simulink model "ConverterControl"  (R2024a)
settings: Solver=FixedStepAuto  StartTime=0.0  StopTime=10.0  FixedStep=0.0001  RelTol=1e-3
model workspace (MAT data in the model file):
  Ts = 0.001
libraries: slpidlib x1
settings Model: Creator=Henrique Mesquita  LastModifiedBy=Henrique Mesquita
settings ModelReferenceCC: EnableParallelModelReferenceBuilds=on  ParallelModelReferenceMATLABWorkerInit=Load Top Model

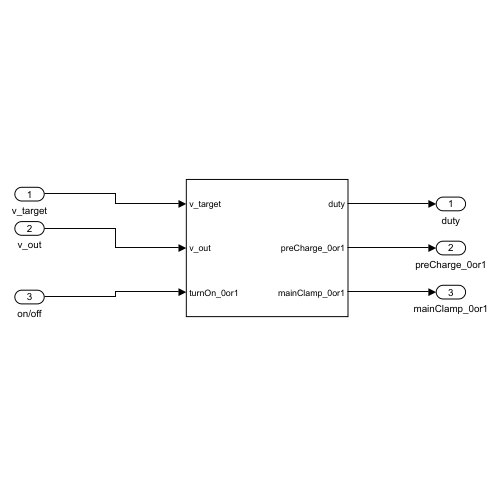
[thumbnail: Simulink's stored preview of the top-level diagram]
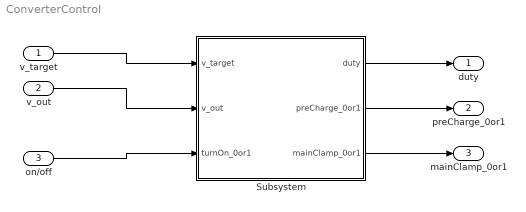
== system ConverterControl ==
  v_target : Inport
  v_out : Inport  Port=2
  on/off : Inport  Port=3
  Subsystem : Subsystem
  duty : Outport
  preCharge_0or1 : Outport  Port=2
  mainClamp_0or1 : Outport  Port=3
  wires:
  v_target/1 -> Subsystem/1(v_target)
  v_out/1 -> Subsystem/2(v_out)
  on/off/1 -> Subsystem/3(turnOn_0or1)
  Subsystem/1(duty) -> duty/1
  Subsystem/2(preCharge_0or1) -> preCharge_0or1/1
  Subsystem/3(mainClamp_0or1) -> mainClamp_0or1/1

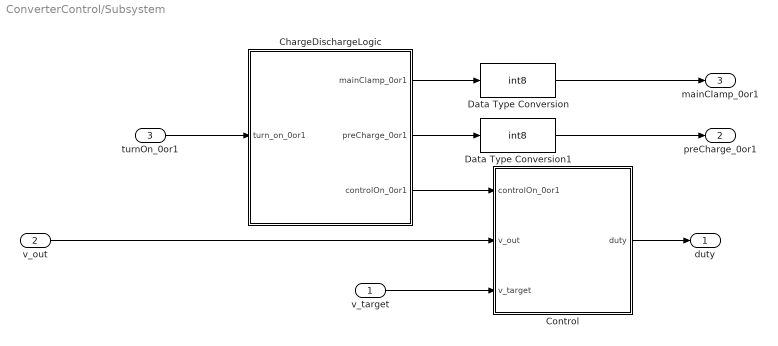
== system ConverterControl/Subsystem ==
  v_target : Inport
  v_out : Inport  Port=2
  turnOn_0or1 : Inport  Port=3
  ChargeDischargeLogic : Stateflow chart  TreatAsAtomicUnit=on
      settings: MinAlgLoopOccurrences=on  PortSchema="{\"entries\":[{\"content\":{\"sides\":[{\"content\":{\"connectorIds\":[\"In1\"]},\"type\":\"ConnectorPlacement.EquallySpacedRectSide\",\"uuid\":\"910d4061-f626-4e59-a733-d82b97cff3cc\"},{\"content\":{\"connectorIds\":[\"Out2\",\"Out3\",\"Out1\"],\"side\":\"RIGHT\"},\"type\":\"ConnectorPlacement.EquallySpacedRectSide\",\"uuid\":\"b59b9408-6f77-4dbd-8f13-72437fb6cf18\"},{\"content\":{\"side\":\"TOP\"},\"type\":\"ConnectorPlacement.EquallySpacedRectSide\",\"uuid\":\"cf8d6f90-ecc3-4087-bd33-4c97bca352fd\"}]},\"type\":\"ConnectorPlacement.EquallySpacedConnector\",\"uuid\":\"df8521dc-5e97-4acd-b29d-9728290d2892\"}],\"packageUris\":[\"http://schema.mathworks.com/mf0/Connector/R2020b\"],\"version\":\"1.0\"}"
  Control : Subsystem
  Data Type Conversion : DataTypeConversion  OutDataTypeStr=int8  SaturateOnIntegerOverflow=off  RndMeth=Floor
  Data Type Conversion1 : DataTypeConversion  OutDataTypeStr=int8  SaturateOnIntegerOverflow=off  RndMeth=Floor
  duty : Outport
  preCharge_0or1 : Outport  Port=2  OutDataTypeStr=int8
  mainClamp_0or1 : Outport  Port=3  OutDataTypeStr=int8
  wires:
  v_target/1 -> Control/3(v_target)
  v_out/1 -> Control/2(v_out)
  ChargeDischargeLogic/1(controlOn_0or1) -> Control/1(controlOn_0or1)
  Control/1(duty) -> duty/1
  turnOn_0or1/1 -> ChargeDischargeLogic/1(turn_on_0or1)
  ChargeDischargeLogic/3(preCharge_0or1) -> Data Type Conversion1/1
  ChargeDischargeLogic/2(mainClamp_0or1) -> Data Type Conversion/1
  Data Type Conversion/1 -> mainClamp_0or1/1
  Data Type Conversion1/1 -> preCharge_0or1/1

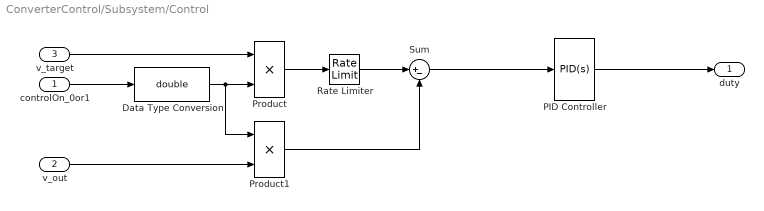
== system ConverterControl/Subsystem/Control ==
  controlOn_0or1 : Inport
  v_out : Inport  Port=2
  v_target : Inport  Port=3
  Data Type Conversion : DataTypeConversion  OutDataTypeStr=double  SaturateOnIntegerOverflow=off  RndMeth=Floor
  PID Controller : slpidlib/PID Controller  Controller=PID  Form=Parallel  TimeDomain=Continuous-time  UseExternalTs=off  SampleTime=-1  IntegratorMethod=Forward Euler  FilterMethod=Forward Euler  ControllerParametersSource=internal  P=0.000137  I=0.512  UseKiTs=off  D=9.21e-09  UseExternalDerivativeSource=off  N=100  UseFilter=on  TunerSelectOption=Transfer Function Based (PID Tuner App)  InitialConditionSource=internal  InitialConditionForIntegrator=0  InitialConditionForFilter=0  DifferentiatorICPrevScaledInput=0  ExternalReset=none  IgnoreLimit=on  TrackingMode=off  Kt=1  LimitOutput=on  SatLimitsSource=internal  UpperSaturationLimit=0.9  LowerSaturationLimit=0  LinearizeAsGain=on  AntiWindupMode=clamping  Kb=1  LimitIntegrator=on  UpperIntegratorSaturationLimit=1  LowerIntegratorSaturationLimit=0  POutMin=[]  POutMax=[]  IOutMin=[]  IOutMax=[]  DOutMin=[]  DOutMax=[]  NOutMin=[]  NOutMax=[]  SumOutMin=[]  SumOutMax=[]  SaturationOutMin=[]  SaturationOutMax=[]  PParamMin=[]  PParamMax=[]  IParamMin=[]  IParamMax=[]  DParamMin=[]  DParamMax=[]  NParamMin=[]  NParamMax=[]  KbParamMin=[]  KbParamMax=[]  KtParamMin=[]  KtParamMax=[]  KbOutMin=[]  KbOutMax=[]  KtOutMin=[]  KtOutMax=[]  IntegratorOutMin=[]  IntegratorOutMax=[]  FilterOutMin=[]  FilterOutMax=[]  SumI1OutMin=[]  SumI1OutMax=[]  SumI2OutMin=[]  SumI2OutMax=[]  SumI3OutMin=[]  SumI3OutMax=[]  SumI4OutMin=[]  SumI4OutMax=[]  SumDOutMin=[]  SumDOutMax=[]  DifferentiatorOutMin=[]  DifferentiatorOutMax=[]  FilterDiffOutCoefMin=[]  FilterDiffOutCoefMax=[]  ReciprocalOutMin=[]  ReciprocalOutMax=[]  SumDenOutMin=[]  SumDenOutMax=[]  SumNumOutMin=[]  SumNumOutMax=[]  DivideOutMin=[]  DivideOutMax=[]  UdiffTsProdOutMin=[]  UdiffTsProdOutMax=[]  NTsProdOutMin=[]  NTsProdOutMax=[]  UintegralTsProdOutMin=[]  UintegralTsProdOutMax=[]  UngainTsProdOutMin=[]  UngainTsProdOutMax=[]  ClampingZeroOutDataTypeStr=Inherit: Inherit via back propagation  ClampingZeroOutMin=[]  ClampingZeroOutMax=[]  FilterDenConstantOutDataTypeStr=Inherit: Inherit via back propagation  FilterDenConstantOutMin=[]  FilterDenConstantOutMax=[]  PCopyOutDataTypeStr=Inherit: Inherit via back propagation  PCopyOutMin=[]  PCopyOutMax=[]  NCopyOutDataTypeStr=Inherit: Inherit via back propagation  NCopyOutMin=[]  NCopyOutMax=[]  IntegratorContinuousStateAttributes=''  IntegratorStateMustResolveToSignalObject=off  IntegratorRTWStateStorageClass=Auto  FilterContinuousStateAttributes=''  FilterStateMustResolveToSignalObject=off  FilterRTWStateStorageClass=Auto  ParallelPVariant=InternalParameters  IdealPVariant=Disabled  IVariant=InternalParameters  DVariant=InternalParameters  IntegratorVariant=Continuous  SatVariant=Enabled  AWVariant=ContClampingParallel  PCopyVariant=Disabled  TRVariant=Disabled  FdbkBlocksVariant=Forward  IdealPFdbkVariant=Disabled  SatFdbkVariant=Disabled  DerivativeFilterVariant=ContFilter  NVariant=InternalParameters  NCopyVariant=Disabled  FilterICVariant=InternalICsFilter  IntegratorICVariant=InternalICs  ExternalResetVariant=Disabled  TRSumVariant=Passthrough  SumFdbkVariant=Disabled  SumVariant=Sum_PID  TsampFilterVariant=InternalTs  TsampNgainVariant=Passthrough  TsampIntegralVariant=Disabled_SignalSpec  ExternalSaturationOutDataTypeStr=Inherit: Same as second input  DerivativeSourceVariant=ErrorSignal
  Product : Product
  Product1 : Product
  Rate Limiter : RateLimiter  RisingSlewLimit=20  FallingSlewLimit=-20
  Sum : Sum  Inputs=|+-
  duty : Outport
  wires:
  controlOn_0or1/1 -> Data Type Conversion/1
  Rate Limiter/1 -> Sum/1
  Sum/1 -> PID Controller/1
  Product/1 -> Rate Limiter/1
  Product1/1 -> Sum/2
  PID Controller/1 -> duty/1
  v_target/1 -> Product/1
  Data Type Conversion/1 -> Product1/1, Product/2
  v_out/1 -> Product1/2

== stateflow chart ConverterControl/Subsystem/ChargeDischargeLogic ==
  settings: stateMachineType=MOORE_MACHINE
  state Converter_off
    preCharge_0or1 = 0;
    mainClamp_0or1 = 0;
    controlOn_0or1 = 0;
  state PreCharge1
    preCharge_0or1 = 1;
  state Converter_on
    controlOn_0or1 = 1;
    preCharge_0or1 = 0;
    mainClamp_0or1 = 1;
  state Discharge
    preCharge_0or1 = 1;
    mainClamp_0or1 = 0;
    controlOn_0or1 = 0;
  (default) -> Converter_off
  PreCharge1 -> Converter_on : after(3,sec)
  Converter_off -> PreCharge1 : [turn_on_0or1 == 1]
  Discharge -> Converter_off : after(10,sec)
  Converter_on -> Discharge : [turn_on_0or1==0]
  data: turn_on_0or1 input boolean; controlOn_0or1 output; mainClamp_0or1 output; preCharge_0or1 output
